simulink model "EAF_simscape"  (R2025b)
settings: Solver=ode23t  StartTime=0.0  StopTime=5  RelTol=1e-3
undefined symbols (not defined in the file or in its folder): Three_PhaseSeriesRLCLoad_class, Three_PhaseSource_class, Three_PhaseTransformer_2_class, Three_PhaseTransformer_T_class, Three_PhaseV_IMeasuremen_class
libraries: ee_lib x12, nesl_utility x9, fl_lib x6, elec_conv_Three_PhaseV_IMeasuremen x4, eeRmsMeasurement x3, elec_conv_sl_RMS x3, spsVariableResistorLib x3, elec_conv_Three_PhaseSeriesRLCBran x3, elec_conv_Three_PhaseSeriesRLCLoad x2, elec_conv_Three_PhaseTransformer_2 x2, elec_conv_Three_PhaseTransformer_T x1, elec_conv_Three_PhaseSource x1
(part 2 of 2)

== system EAF_simscape/Three-Phase Transformer (Two Windings) ==
  Two-Winding Transformer (Three-Phase) : ee_lib/Passive/Transformers/Two-Winding Transformer (Three-Phase)  SRated=250000000 V*A  FRated=60 Hz  Winding1Connection=3  VRated1=35000 V  Winding2Connection=3  VRated2=420.02 V  CoreType=2  pu_Rw1=Three_PhaseTransformer_2_class('Yg','Yg','pu',[250000000 60],[35000 6.9e-05 2.2e-06],[420.02 6.9e-05 2.2e-06],500,500,0.5,[0 0;0.0024 1.2;1 1.52],[0.8 -0.8 0.7],'off','off').objParamMappingDerived.NewDerivedParam.pu_Rw1  pu_Rw2=Three_PhaseTransformer_2_class('Yg','Yg','pu',[250000000 60],[35000 6.9e-05 2.2e-06],[420.02 6.9e-05 2.2e-06],500,500,0.5,[0 0;0.0024 1.2;1 1.52],[0.8 -0.8 0.7],'off','off').objParamMappingDerived.NewDerivedParam.pu_Rw2  leakage_reactance_option=ee.enum.transformer_leakage.include  pu_Xl1=Three_PhaseTransformer_2_class('Yg','Yg','pu',[250000000 60],[35000 6.9e-05 2.2e-06],[420.02 6.9e-05 2.2e-06],500,500,0.5,[0 0;0.0024 1.2;1 1.52],[0.8 -0.8 0.7],'off','off').objParamMappingDerived.NewDerivedParam.pu_Xl1  pu_Xl2=Three_PhaseTransformer_2_class('Yg','Yg','pu',[250000000 60],[35000 6.9e-05 2.2e-06],[420.02 6.9e-05 2.2e-06],500,500,0.5,[0 0;0.0024 1.2;1 1.52],[0.8 -0.8 0.7],'off','off').objParamMappingDerived.NewDerivedParam.pu_Xl2  magnetizing_resistance_option=ee.enum.transformer_magnetizingResistance.include  pu_Rm=Three_PhaseTransformer_2_class('Yg','Yg','pu',[250000000 60],[35000 6.9e-05 2.2e-06],[420.02 6.9e-05 2.2e-06],500,500,0.5,[0 0;0.0024 1.2;1 1.52],[0.8 -0.8 0.7],'off','off').objParamMappingDerived.NewDerivedParam.pu_Rm  magnetizing_reactance_option=ee.enum.transformer_magnetizingReactance.include  saturation_option=1  pu_Xm=Three_PhaseTransformer_2_class('Yg','Yg','pu',[250000000 60],[35000 6.9e-05 2.2e-06],[420.02 6.9e-05 2.2e-06],500,500,0.5,[0 0;0.0024 1.2;1 1.52],[0.8 -0.8 0.7],'off','off').objParamMappingDerived.NewDerivedParam.pu_Xm  current_data=Three_PhaseTransformer_2_class('Yg','Yg','pu',[250000000 60],[35000 6.9e-05 2.2e-06],[420.02 6.9e-05 2.2e-06],500,500,0.5,[0 0;0.0024 1.2;1 1.52],[0.8 -0.8 0.7],'off','off').objParamMappingDerived.NewDerivedParam.current_data  magnetic_flux_data=Three_PhaseTransformer_2_class('Yg','Yg','pu',[250000000 60],[35000 6.9e-05 2.2e-06],[420.02 6.9e-05 2.2e-06],500,500,0.5,[0 0;0.0024 1.2;1 1.52],[0.8 -0.8 0.7],'off','off').objParamMappingDerived.NewDerivedParam.magnetic_flux_data  pu_X0=Three_PhaseTransformer_2_class('Yg','Yg','pu',[250000000 60],[35000 6.9e-05 2.2e-06],[420.02 6.9e-05 2.2e-06],500,500,0.5,[0 0;0.0024 1.2;1 1.52],[0.8 -0.8 0.7],'off','off').objParamMappingDerived.NewDerivedParam.pu_X0  i1_specify=off  i1_priority=None  i1=[ 0 0 0 ] A  i1_nominal_specify=off  i1_nominal_value=1  i1_nominal_unit=A  i2_specify=off  i2_priority=None  i2=[ 0 0 0 ] A  i2_nominal_specify=off  i2_nominal_value=1  i2_nominal_unit=A  phi_specify=off  phi_priority=None  phi=Three_PhaseTransformer_2_class('Yg','Yg','pu',[250000000 60],[35000 6.9e-05 2.2e-06],[420.02 6.9e-05 2.2e-06],500,500,0.5,[0 0;0.0024 1.2;1 1.52],[0.8 -0.8 0.7],'off','off').objParamMappingDerived.NewDerivedParam.phi  phi_nominal_specify=off  phi_nominal_value=1  phi_nominal_unit=1  power_dissipated_specify=off  power_dissipated_priority=None  power_dissipated=0 W  power_dissipated_nominal_specify=off  power_dissipated_nominal_value=1  power_dissipated_nominal_unit=W
      settings: InternalSimscapePortConfiguration="{\"Bottom\":[],\"Left\":[{\"id\":\"a1\",\"label\":\"a1\",\"type\":\"foundation.electrical.electrical\"},{\"id\":\"b1\",\"label\":\"b1\",\"type\":\"foundation.electrical.electrical\"},{\"id\":\"c1\",\"label\":\"c1\",\"type\":\"foundation.electrical.electrical\"}],\"Right\":[{\"id\":\"a2\",\"label\":\"a2\",\"type\":\"foundation.electrical.electrical\"},{\"id\":\"b2\",\"label\":\"b2\",\"type\":\"foundation.electrical.electrical\"},{\"id\":\"c2\",\"label\":\"c2\",\"type\":\"foundation.electrical.electrical\"}],\"Top\":[]}"
  A : PMIOPort  Side=Left
  B : PMIOPort  Port=2  Side=Left
  C : PMIOPort  Port=3  Side=Left
  a : PMIOPort  Port=4  Side=Right
  b : PMIOPort  Port=5  Side=Right
  c : PMIOPort  Port=6  Side=Right
  connections:
  A/RConn1 -- Two-Winding Transformer (Three-Phase)/LConn1
  B/RConn1 -- Two-Winding Transformer (Three-Phase)/LConn2
  C/RConn1 -- Two-Winding Transformer (Three-Phase)/LConn3
  Two-Winding Transformer (Three-Phase)/RConn3 -- c/RConn1
  Two-Winding Transformer (Three-Phase)/RConn1 -- a/RConn1
  Two-Winding Transformer (Three-Phase)/RConn2 -- b/RConn1

== system EAF_simscape/Three-Phase Transformer (Two Windings)1 ==
  Two-Winding Transformer (Three-Phase) : ee_lib/Passive/Transformers/Two-Winding Transformer (Three-Phase)  SRated=250000000 V*A  FRated=60 Hz  Winding1Connection=3  VRated1=735000 V  Winding2Connection=3  VRated2=8820 V  CoreType=2  pu_Rw1=Three_PhaseTransformer_2_class('Yg','Yg','pu',[250000000 60],[735000 6.9e-05 2.2e-06],[8820 6.9e-05 2.2e-06],500,500,0.5,[0 0;0.0024 1.2;1 1.52],[0.8 -0.8 0.7],'off','off').objParamMappingDerived.NewDerivedParam.pu_Rw1  pu_Rw2=Three_PhaseTransformer_2_class('Yg','Yg','pu',[250000000 60],[735000 6.9e-05 2.2e-06],[8820 6.9e-05 2.2e-06],500,500,0.5,[0 0;0.0024 1.2;1 1.52],[0.8 -0.8 0.7],'off','off').objParamMappingDerived.NewDerivedParam.pu_Rw2  leakage_reactance_option=ee.enum.transformer_leakage.include  pu_Xl1=Three_PhaseTransformer_2_class('Yg','Yg','pu',[250000000 60],[735000 6.9e-05 2.2e-06],[8820 6.9e-05 2.2e-06],500,500,0.5,[0 0;0.0024 1.2;1 1.52],[0.8 -0.8 0.7],'off','off').objParamMappingDerived.NewDerivedParam.pu_Xl1  pu_Xl2=Three_PhaseTransformer_2_class('Yg','Yg','pu',[250000000 60],[735000 6.9e-05 2.2e-06],[8820 6.9e-05 2.2e-06],500,500,0.5,[0 0;0.0024 1.2;1 1.52],[0.8 -0.8 0.7],'off','off').objParamMappingDerived.NewDerivedParam.pu_Xl2  magnetizing_resistance_option=ee.enum.transformer_magnetizingResistance.include  pu_Rm=Three_PhaseTransformer_2_class('Yg','Yg','pu',[250000000 60],[735000 6.9e-05 2.2e-06],[8820 6.9e-05 2.2e-06],500,500,0.5,[0 0;0.0024 1.2;1 1.52],[0.8 -0.8 0.7],'off','off').objParamMappingDerived.NewDerivedParam.pu_Rm  magnetizing_reactance_option=ee.enum.transformer_magnetizingReactance.include  saturation_option=1  pu_Xm=Three_PhaseTransformer_2_class('Yg','Yg','pu',[250000000 60],[735000 6.9e-05 2.2e-06],[8820 6.9e-05 2.2e-06],500,500,0.5,[0 0;0.0024 1.2;1 1.52],[0.8 -0.8 0.7],'off','off').objParamMappingDerived.NewDerivedParam.pu_Xm  current_data=Three_PhaseTransformer_2_class('Yg','Yg','pu',[250000000 60],[735000 6.9e-05 2.2e-06],[8820 6.9e-05 2.2e-06],500,500,0.5,[0 0;0.0024 1.2;1 1.52],[0.8 -0.8 0.7],'off','off').objParamMappingDerived.NewDerivedParam.current_data  magnetic_flux_data=Three_PhaseTransformer_2_class('Yg','Yg','pu',[250000000 60],[735000 6.9e-05 2.2e-06],[8820 6.9e-05 2.2e-06],500,500,0.5,[0 0;0.0024 1.2;1 1.52],[0.8 -0.8 0.7],'off','off').objParamMappingDerived.NewDerivedParam.magnetic_flux_data  pu_X0=Three_PhaseTransformer_2_class('Yg','Yg','pu',[250000000 60],[735000 6.9e-05 2.2e-06],[8820 6.9e-05 2.2e-06],500,500,0.5,[0 0;0.0024 1.2;1 1.52],[0.8 -0.8 0.7],'off','off').objParamMappingDerived.NewDerivedParam.pu_X0  i1_specify=off  i1_priority=None  i1=[ 0 0 0 ] A  i1_nominal_specify=off  i1_nominal_value=1  i1_nominal_unit=A  i2_specify=off  i2_priority=None  i2=[ 0 0 0 ] A  i2_nominal_specify=off  i2_nominal_value=1  i2_nominal_unit=A  phi_specify=off  phi_priority=None  phi=Three_PhaseTransformer_2_class('Yg','Yg','pu',[250000000 60],[735000 6.9e-05 2.2e-06],[8820 6.9e-05 2.2e-06],500,500,0.5,[0 0;0.0024 1.2;1 1.52],[0.8 -0.8 0.7],'off','off').objParamMappingDerived.NewDerivedParam.phi  phi_nominal_specify=off  phi_nominal_value=1  phi_nominal_unit=1  power_dissipated_specify=off  power_dissipated_priority=None  power_dissipated=0 W  power_dissipated_nominal_specify=off  power_dissipated_nominal_value=1  power_dissipated_nominal_unit=W
      settings: InternalSimscapePortConfiguration="{\"Bottom\":[],\"Left\":[{\"id\":\"a1\",\"label\":\"a1\",\"type\":\"foundation.electrical.electrical\"},{\"id\":\"b1\",\"label\":\"b1\",\"type\":\"foundation.electrical.electrical\"},{\"id\":\"c1\",\"label\":\"c1\",\"type\":\"foundation.electrical.electrical\"}],\"Right\":[{\"id\":\"a2\",\"label\":\"a2\",\"type\":\"foundation.electrical.electrical\"},{\"id\":\"b2\",\"label\":\"b2\",\"type\":\"foundation.electrical.electrical\"},{\"id\":\"c2\",\"label\":\"c2\",\"type\":\"foundation.electrical.electrical\"}],\"Top\":[]}"
  A : PMIOPort  Side=Left
  B : PMIOPort  Port=2  Side=Left
  C : PMIOPort  Port=3  Side=Left
  a : PMIOPort  Port=4  Side=Right
  b : PMIOPort  Port=5  Side=Right
  c : PMIOPort  Port=6  Side=Right
  connections:
  A/RConn1 -- Two-Winding Transformer (Three-Phase)/LConn1
  B/RConn1 -- Two-Winding Transformer (Three-Phase)/LConn2
  C/RConn1 -- Two-Winding Transformer (Three-Phase)/LConn3
  Two-Winding Transformer (Three-Phase)/RConn3 -- c/RConn1
  Two-Winding Transformer (Three-Phase)/RConn1 -- a/RConn1
  Two-Winding Transformer (Three-Phase)/RConn2 -- b/RConn1

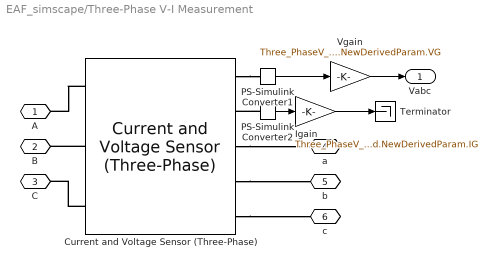
== system EAF_simscape/Three-Phase V-I Measurement ==
  Current and Voltage Sensor (Three-Phase) : ee_lib/Sensors & Transducers/Current and Voltage Sensor (Three-Phase)  vMeasurementType=1  outputUnit=2  SRated=100000000 V*A  VRated=500000 V  I_specify=off  I_priority=None  I=[ 0 0 0 ] A  I_nominal_specify=off  I_nominal_value=1  I_nominal_unit=A  V_specify=off  V_priority=None  V=[ 0 0 0 ] V  V_nominal_specify=off  V_nominal_value=1  V_nominal_unit=V
      settings: InternalSimscapePortConfiguration="{\"Bottom\":[],\"Left\":[{\"id\":\"a1\",\"label\":\"a1\",\"type\":\"foundation.electrical.electrical\"},{\"id\":\"b1\",\"label\":\"b1\",\"type\":\"foundation.electrical.electrical\"},{\"id\":\"c1\",\"label\":\"c1\",\"type\":\"foundation.electrical.electrical\"}],\"Right\":[{\"id\":\"V_output\",\"label\":\"V\",\"type\":\"output\"},{\"id\":\"I_output\",\"label\":\"I\",\"type\":\"output\"},{\"id\":\"a2\",\"label\":\"a2\",\"type\":\"foundation.electrical.electrical\"},{\"id\":\"b2\",\"label\":\"b2\",\"type\":\"foundation.electrical.electrical\"},{\"id\":\"c2\",\"label\":\"c2\",\"type\":\"foundation.electrical.electrical\"}],\"Top\":[]}"
  Igain : Gain  Gain=Three_PhaseV_IMeasuremen_class('phase-to-phase','no','off','off','off',100000000,500000).objParamMappingDerived.NewDerivedParam.IG
  PS-Simulink Converter1 : nesl_utility/PS-Simulink Converter  PhysicalDomain=network_engine_domain  SubClassName=ps_output  LeftPortType=input  RightPortType=output  PseudoPeriodic=off  Frequencies=[]  VectorFormat=1-D array  Unit=1  AffineConversion=off
  PS-Simulink Converter2 : nesl_utility/PS-Simulink Converter  PhysicalDomain=network_engine_domain  SubClassName=ps_output  LeftPortType=input  RightPortType=output  PseudoPeriodic=off  Frequencies=[]  VectorFormat=1-D array  Unit=1  AffineConversion=off
  Terminator : Terminator
  Vgain : Gain  Gain=Three_PhaseV_IMeasuremen_class('phase-to-phase','no','off','off','off',100000000,500000).objParamMappingDerived.NewDerivedParam.VG
  A : PMIOPort  Side=Left
  B : PMIOPort  Port=2  Side=Left
  C : PMIOPort  Port=3  Side=Left
  a : PMIOPort  Port=4  Side=Right
  b : PMIOPort  Port=5  Side=Right
  c : PMIOPort  Port=6  Side=Right
  Vabc : Outport  VectorParamsAs1DForOutWhenUnconnected=off
  wires:
  Igain/1 -> Terminator/1
  PS-Simulink Converter2/1 -> Igain/1
  Vgain/1 -> Vabc/1
  PS-Simulink Converter1/1 -> Vgain/1
  connections:
  PS-Simulink Converter2/LConn1 -- Current and Voltage Sensor (Three-Phase)/RConn2
  Current and Voltage Sensor (Three-Phase)/RConn1 -- PS-Simulink Converter1/LConn1
  Current and Voltage Sensor (Three-Phase)/LConn2 -- B/RConn1
  Current and Voltage Sensor (Three-Phase)/LConn1 -- A/RConn1
  Current and Voltage Sensor (Three-Phase)/LConn3 -- C/RConn1
  Current and Voltage Sensor (Three-Phase)/RConn3 -- a/RConn1
  Current and Voltage Sensor (Three-Phase)/RConn4 -- b/RConn1
  Current and Voltage Sensor (Three-Phase)/RConn5 -- c/RConn1

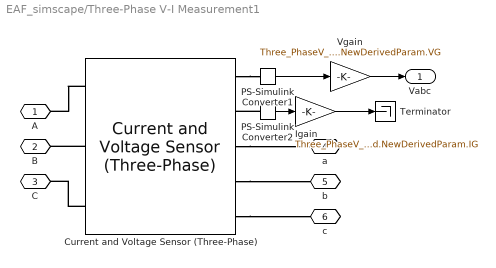
== system EAF_simscape/Three-Phase V-I Measurement1 ==
  Current and Voltage Sensor (Three-Phase) : ee_lib/Sensors & Transducers/Current and Voltage Sensor (Three-Phase)  vMeasurementType=1  outputUnit=2  SRated=100000000 V*A  VRated=500000 V  I_specify=off  I_priority=None  I=[ 0 0 0 ] A  I_nominal_specify=off  I_nominal_value=1  I_nominal_unit=A  V_specify=off  V_priority=None  V=[ 0 0 0 ] V  V_nominal_specify=off  V_nominal_value=1  V_nominal_unit=V
      settings: InternalSimscapePortConfiguration="{\"Bottom\":[],\"Left\":[{\"id\":\"a1\",\"label\":\"a1\",\"type\":\"foundation.electrical.electrical\"},{\"id\":\"b1\",\"label\":\"b1\",\"type\":\"foundation.electrical.electrical\"},{\"id\":\"c1\",\"label\":\"c1\",\"type\":\"foundation.electrical.electrical\"}],\"Right\":[{\"id\":\"V_output\",\"label\":\"V\",\"type\":\"output\"},{\"id\":\"I_output\",\"label\":\"I\",\"type\":\"output\"},{\"id\":\"a2\",\"label\":\"a2\",\"type\":\"foundation.electrical.electrical\"},{\"id\":\"b2\",\"label\":\"b2\",\"type\":\"foundation.electrical.electrical\"},{\"id\":\"c2\",\"label\":\"c2\",\"type\":\"foundation.electrical.electrical\"}],\"Top\":[]}"
  Igain : Gain  Gain=Three_PhaseV_IMeasuremen_class('phase-to-phase','no','off','off','off',100000000,500000).objParamMappingDerived.NewDerivedParam.IG
  PS-Simulink Converter1 : nesl_utility/PS-Simulink Converter  PhysicalDomain=network_engine_domain  SubClassName=ps_output  LeftPortType=input  RightPortType=output  PseudoPeriodic=off  Frequencies=[]  VectorFormat=1-D array  Unit=1  AffineConversion=off
  PS-Simulink Converter2 : nesl_utility/PS-Simulink Converter  PhysicalDomain=network_engine_domain  SubClassName=ps_output  LeftPortType=input  RightPortType=output  PseudoPeriodic=off  Frequencies=[]  VectorFormat=1-D array  Unit=1  AffineConversion=off
  Terminator : Terminator
  Vgain : Gain  Gain=Three_PhaseV_IMeasuremen_class('phase-to-phase','no','off','off','off',100000000,500000).objParamMappingDerived.NewDerivedParam.VG
  A : PMIOPort  Side=Left
  B : PMIOPort  Port=2  Side=Left
  C : PMIOPort  Port=3  Side=Left
  a : PMIOPort  Port=4  Side=Right
  b : PMIOPort  Port=5  Side=Right
  c : PMIOPort  Port=6  Side=Right
  Vabc : Outport  VectorParamsAs1DForOutWhenUnconnected=off
  wires:
  Igain/1 -> Terminator/1
  PS-Simulink Converter2/1 -> Igain/1
  Vgain/1 -> Vabc/1
  PS-Simulink Converter1/1 -> Vgain/1
  connections:
  PS-Simulink Converter2/LConn1 -- Current and Voltage Sensor (Three-Phase)/RConn2
  Current and Voltage Sensor (Three-Phase)/RConn1 -- PS-Simulink Converter1/LConn1
  Current and Voltage Sensor (Three-Phase)/LConn2 -- B/RConn1
  Current and Voltage Sensor (Three-Phase)/LConn1 -- A/RConn1
  Current and Voltage Sensor (Three-Phase)/LConn3 -- C/RConn1
  Current and Voltage Sensor (Three-Phase)/RConn3 -- a/RConn1
  Current and Voltage Sensor (Three-Phase)/RConn4 -- b/RConn1
  Current and Voltage Sensor (Three-Phase)/RConn5 -- c/RConn1

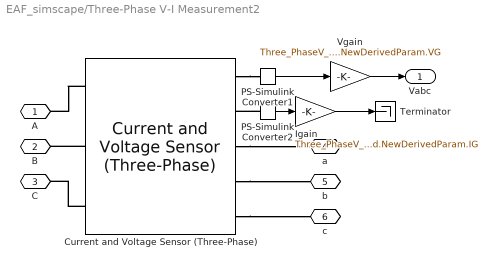
== system EAF_simscape/Three-Phase V-I Measurement2 ==
  Current and Voltage Sensor (Three-Phase) : ee_lib/Sensors & Transducers/Current and Voltage Sensor (Three-Phase)  vMeasurementType=1  outputUnit=2  SRated=100000000 V*A  VRated=500000 V  I_specify=off  I_priority=None  I=[ 0 0 0 ] A  I_nominal_specify=off  I_nominal_value=1  I_nominal_unit=A  V_specify=off  V_priority=None  V=[ 0 0 0 ] V  V_nominal_specify=off  V_nominal_value=1  V_nominal_unit=V
      settings: InternalSimscapePortConfiguration="{\"Bottom\":[],\"Left\":[{\"id\":\"a1\",\"label\":\"a1\",\"type\":\"foundation.electrical.electrical\"},{\"id\":\"b1\",\"label\":\"b1\",\"type\":\"foundation.electrical.electrical\"},{\"id\":\"c1\",\"label\":\"c1\",\"type\":\"foundation.electrical.electrical\"}],\"Right\":[{\"id\":\"V_output\",\"label\":\"V\",\"type\":\"output\"},{\"id\":\"I_output\",\"label\":\"I\",\"type\":\"output\"},{\"id\":\"a2\",\"label\":\"a2\",\"type\":\"foundation.electrical.electrical\"},{\"id\":\"b2\",\"label\":\"b2\",\"type\":\"foundation.electrical.electrical\"},{\"id\":\"c2\",\"label\":\"c2\",\"type\":\"foundation.electrical.electrical\"}],\"Top\":[]}"
  Igain : Gain  Gain=Three_PhaseV_IMeasuremen_class('phase-to-phase','no','off','off','off',100000000,500000).objParamMappingDerived.NewDerivedParam.IG
  PS-Simulink Converter1 : nesl_utility/PS-Simulink Converter  PhysicalDomain=network_engine_domain  SubClassName=ps_output  LeftPortType=input  RightPortType=output  PseudoPeriodic=off  Frequencies=[]  VectorFormat=1-D array  Unit=1  AffineConversion=off
  PS-Simulink Converter2 : nesl_utility/PS-Simulink Converter  PhysicalDomain=network_engine_domain  SubClassName=ps_output  LeftPortType=input  RightPortType=output  PseudoPeriodic=off  Frequencies=[]  VectorFormat=1-D array  Unit=1  AffineConversion=off
  Terminator : Terminator
  Vgain : Gain  Gain=Three_PhaseV_IMeasuremen_class('phase-to-phase','no','off','off','off',100000000,500000).objParamMappingDerived.NewDerivedParam.VG
  A : PMIOPort  Side=Left
  B : PMIOPort  Port=2  Side=Left
  C : PMIOPort  Port=3  Side=Left
  a : PMIOPort  Port=4  Side=Right
  b : PMIOPort  Port=5  Side=Right
  c : PMIOPort  Port=6  Side=Right
  Vabc : Outport  VectorParamsAs1DForOutWhenUnconnected=off
  wires:
  Igain/1 -> Terminator/1
  PS-Simulink Converter2/1 -> Igain/1
  Vgain/1 -> Vabc/1
  PS-Simulink Converter1/1 -> Vgain/1
  connections:
  PS-Simulink Converter2/LConn1 -- Current and Voltage Sensor (Three-Phase)/RConn2
  Current and Voltage Sensor (Three-Phase)/RConn1 -- PS-Simulink Converter1/LConn1
  Current and Voltage Sensor (Three-Phase)/LConn2 -- B/RConn1
  Current and Voltage Sensor (Three-Phase)/LConn1 -- A/RConn1
  Current and Voltage Sensor (Three-Phase)/LConn3 -- C/RConn1
  Current and Voltage Sensor (Three-Phase)/RConn3 -- a/RConn1
  Current and Voltage Sensor (Three-Phase)/RConn4 -- b/RConn1
  Current and Voltage Sensor (Three-Phase)/RConn5 -- c/RConn1

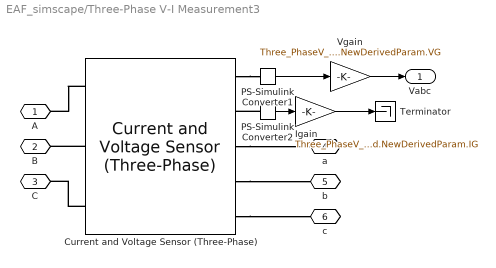
== system EAF_simscape/Three-Phase V-I Measurement3 ==
  Current and Voltage Sensor (Three-Phase) : ee_lib/Sensors & Transducers/Current and Voltage Sensor (Three-Phase)  vMeasurementType=2  outputUnit=2  SRated=100000000 V*A  VRated=500000 V  I_specify=off  I_priority=None  I=[ 0 0 0 ] A  I_nominal_specify=off  I_nominal_value=1  I_nominal_unit=A  V_specify=off  V_priority=None  V=[ 0 0 0 ] V  V_nominal_specify=off  V_nominal_value=1  V_nominal_unit=V
      settings: InternalSimscapePortConfiguration="{\"Bottom\":[],\"Left\":[{\"id\":\"a1\",\"label\":\"a1\",\"type\":\"foundation.electrical.electrical\"},{\"id\":\"b1\",\"label\":\"b1\",\"type\":\"foundation.electrical.electrical\"},{\"id\":\"c1\",\"label\":\"c1\",\"type\":\"foundation.electrical.electrical\"}],\"Right\":[{\"id\":\"V_output\",\"label\":\"V\",\"type\":\"output\"},{\"id\":\"I_output\",\"label\":\"I\",\"type\":\"output\"},{\"id\":\"a2\",\"label\":\"a2\",\"type\":\"foundation.electrical.electrical\"},{\"id\":\"b2\",\"label\":\"b2\",\"type\":\"foundation.electrical.electrical\"},{\"id\":\"c2\",\"label\":\"c2\",\"type\":\"foundation.electrical.electrical\"}],\"Top\":[]}"
  Igain : Gain  Gain=Three_PhaseV_IMeasuremen_class('phase-to-ground','no','off','off','off',100000000,500000).objParamMappingDerived.NewDerivedParam.IG
  PS-Simulink Converter1 : nesl_utility/PS-Simulink Converter  PhysicalDomain=network_engine_domain  SubClassName=ps_output  LeftPortType=input  RightPortType=output  PseudoPeriodic=off  Frequencies=[]  VectorFormat=1-D array  Unit=1  AffineConversion=off
  PS-Simulink Converter2 : nesl_utility/PS-Simulink Converter  PhysicalDomain=network_engine_domain  SubClassName=ps_output  LeftPortType=input  RightPortType=output  PseudoPeriodic=off  Frequencies=[]  VectorFormat=1-D array  Unit=1  AffineConversion=off
  Terminator : Terminator
  Vgain : Gain  Gain=Three_PhaseV_IMeasuremen_class('phase-to-ground','no','off','off','off',100000000,500000).objParamMappingDerived.NewDerivedParam.VG
  A : PMIOPort  Side=Left
  B : PMIOPort  Port=2  Side=Left
  C : PMIOPort  Port=3  Side=Left
  a : PMIOPort  Port=4  Side=Right
  b : PMIOPort  Port=5  Side=Right
  c : PMIOPort  Port=6  Side=Right
  Vabc : Outport  VectorParamsAs1DForOutWhenUnconnected=off
  wires:
  Igain/1 -> Terminator/1
  PS-Simulink Converter2/1 -> Igain/1
  Vgain/1 -> Vabc/1
  PS-Simulink Converter1/1 -> Vgain/1
  connections:
  PS-Simulink Converter2/LConn1 -- Current and Voltage Sensor (Three-Phase)/RConn2
  Current and Voltage Sensor (Three-Phase)/RConn1 -- PS-Simulink Converter1/LConn1
  Current and Voltage Sensor (Three-Phase)/LConn2 -- B/RConn1
  Current and Voltage Sensor (Three-Phase)/LConn1 -- A/RConn1
  Current and Voltage Sensor (Three-Phase)/LConn3 -- C/RConn1
  Current and Voltage Sensor (Three-Phase)/RConn3 -- a/RConn1
  Current and Voltage Sensor (Three-Phase)/RConn4 -- b/RConn1
  Current and Voltage Sensor (Three-Phase)/RConn5 -- c/RConn1

== system EAF_simscape/Three-Phase Source ==
  Electrical Reference : fl_lib/Electrical/Electrical Elements/Electrical Reference
  Voltage Source : ee_lib/Sources/Voltage Source (Three-Phase)  vline_rms=110000 V  shift=0 deg  freq=60 Hz  impedance_option=4  SShortCircuit=100000000 V*A  XR=7  R=Three_PhaseSource_class(110000,60,1.186,0.01658,100000000,110000,7,'on','off').objParamMappingDerived.NewDerivedParam.R Ohm  L=Three_PhaseSource_class(110000,60,1.186,0.01658,100000000,110000,7,'on','off').objParamMappingDerived.NewDerivedParam.L H  harmonic_option=0  harmonic_orders=[5, 7, 11, 13]  harmonic_ratios=[.1, .1, .1, .1]  G_parasitic=0 1/Ohm  I_specify=off  I_priority=None  I=[ 0 0 0 ] A  I_nominal_specify=off  I_nominal_value=1  I_nominal_unit=A
      settings: InternalSimscapePortConfiguration="{\"Bottom\":[],\"Left\":[{\"id\":\"n\",\"label\":\"n\",\"type\":\"foundation.electrical.electrical\"}],\"Right\":[{\"id\":\"a\",\"label\":\"a\",\"type\":\"foundation.electrical.electrical\"},{\"id\":\"b\",\"label\":\"b\",\"type\":\"foundation.electrical.electrical\"},{\"id\":\"c\",\"label\":\"c\",\"type\":\"foundation.electrical.electrical\"}],\"Top\":[]}"
  A : PMIOPort  Side=Right
  B : PMIOPort  Port=2  Side=Right
  C : PMIOPort  Port=3  Side=Right
  connections:
  Voltage Source/RConn2 -- B/RConn1
  Voltage Source/RConn1 -- A/RConn1
  Voltage Source/RConn3 -- C/RConn1
  Electrical Reference/LConn1 -- Voltage Source/LConn1

== system EAF_simscape/Subsystem/Series RLC Branch ==
  Resistor : fl_lib/Electrical/Electrical Elements/Resistor  R=100000 Ohm  i_specify=off  i_priority=None  i=0 A  i_nominal_specify=off  i_nominal_value=1  i_nominal_unit=A  v_specify=off  v_priority=None  v=0 V  v_nominal_specify=off  v_nominal_value=1  v_nominal_unit=V
  + : PMIOPort  Side=Left
  - : PMIOPort  Port=2  Side=Right
  connections:
  +/RConn1 -- Resistor/LConn1
  -/RConn1 -- Resistor/RConn1

== system EAF_simscape/Subsystem1/Series RLC Branch ==
  Resistor : fl_lib/Electrical/Electrical Elements/Resistor  R=100000 Ohm  i_specify=off  i_priority=None  i=0 A  i_nominal_specify=off  i_nominal_value=1  i_nominal_unit=A  v_specify=off  v_priority=None  v=0 V  v_nominal_specify=off  v_nominal_value=1  v_nominal_unit=V
  + : PMIOPort  Side=Left
  - : PMIOPort  Port=2  Side=Right
  connections:
  +/RConn1 -- Resistor/LConn1
  -/RConn1 -- Resistor/RConn1

== system EAF_simscape/Subsystem2/Series RLC Branch ==
  Resistor : fl_lib/Electrical/Electrical Elements/Resistor  R=100000 Ohm  i_specify=off  i_priority=None  i=0 A  i_nominal_specify=off  i_nominal_value=1  i_nominal_unit=A  v_specify=off  v_priority=None  v=0 V  v_nominal_specify=off  v_nominal_value=1  v_nominal_unit=V
  + : PMIOPort  Side=Left
  - : PMIOPort  Port=2  Side=Right
  connections:
  +/RConn1 -- Resistor/LConn1
  -/RConn1 -- Resistor/RConn1
